simulink model "am_modulation_simulink"  (R2015a)
settings: Solver=ode45  StartTime=0.0  StopTime=8  RelTol=1e-3
libraries: commanapbnd3 x1
settings Model: Creator=OSAMA  LastModifiedBy=OSAMA

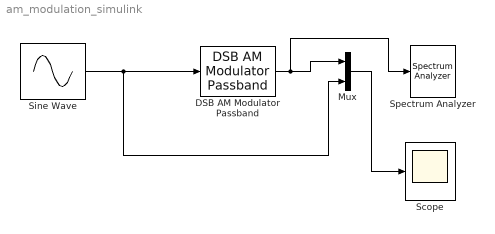
== system am_modulation_simulink ==
  DSB AM Modulator Passband : commanapbnd3/DSB AM Modulator Passband  Fc=300  Ph=0  Offset=0
  Mux : Mux  Inputs=2
  Scope : Scope
      settings: ShowLegends=on
  Sine Wave : Sin  Amplitude=2  Frequency=3  SampleTime=0.001
  Spectrum Analyzer : SpectrumAnalyzer
  wires:
  Sine Wave/1 -> Mux/2, DSB AM Modulator Passband/1
  DSB AM Modulator Passband/1 -> Spectrum Analyzer/1, Mux/1
  Mux/1 -> Scope/1
